simulink library "libreria"  (R2017a)
settings: Solver=VariableStepAuto  StartTime=0.0  StopTime=10.0  RelTol=1e-3
undefined symbols (not defined in the file or in its folder): codertarget, DiscIntNeverNeededParam, gcbh, K, K_PWM, R, Vu, W
libraries: legoev3lib x10, simulink_extras x3, simulink x2
settings Model: Creator=ruben  LastModifiedBy=ruben

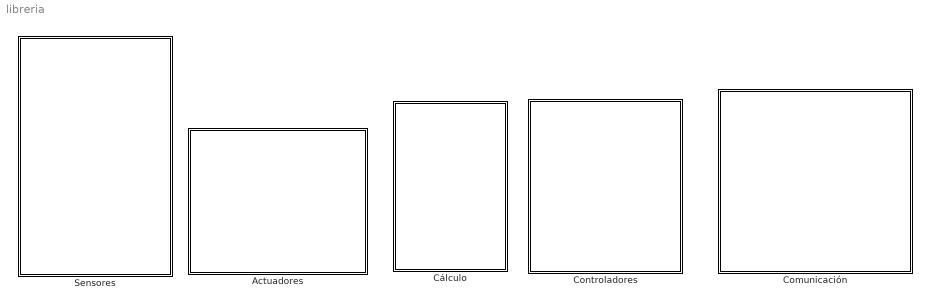
== system libreria ==
  Actuadores : Subsystem
  Comunicación : Subsystem
  Controladores : Subsystem
  Cálculo : Subsystem
  Sensores : Subsystem

== system libreria/Actuadores ==
  Motores : Subsystem  mask(Actuador){}
      mask help:
      | Bloque para la alimentación de los motores en conjunto.
      |
      | Una entrada. Rango de potencia -100/100.
      mask Help:
      | Conexión de entradas:
      | 
      | 	-  Entrada A: Motor izquierdo.
      | 
      | 	- Entrada B: Motor derecho.
      | 
      | Contiene una ganancia para compensar la diferencia existente en la rotación de los motores, explicada en la memoria.
      | 
      | Posibilidad de alimentar cada motor independientemente.
      mask Display: image('D:\RUBEN\Uni\Grado\TFG\Imagenes\Legos\Libreria\motor.png');
  Motores equilibrio : Subsystem  mask(Actuador){}
      mask help:
      | Bloque para la alimentación de los motores en conjunto.
      |
      | Una entrada. Rango de potencia -100/100.
      mask Help:
      | Conexión de entradas:
      | 
      | 	-  Entrada A: Motor izquierdo.
      | 
      | 	- Entrada B: Motor derecho.
      | 
      | Contiene una ganancia para compensar la diferencia existente en la rotación de los motores, explicada en la memoria.
      | 
      | Posibilidad de alimentar cada motor independientemente.
      mask Display: image('D:\RUBEN\Uni\Grado\TFG\Imagenes\Legos\Libreria\motor.png');
  Motores independientes : Subsystem  mask(Actuador){}
      mask help:
      | Bloque para la alimentación de los motores de manera independiente.
      |
      | Dos entradas. Rango de potencia -100/100.
      mask Help:
      | - Puerto A: Motor izquierdo.
      | 
      | - Puerto B: Motor derecho.
      mask Display: image('C:\Users\ruben\Desktop\Eloy\izqu.png');

== system libreria/Comunicación ==
  UDP Envío : S-Function  AncestorBlock=legoev3lib/UDP Send  InitFcn=codertarget.linux.blocks.validateUDPBlock(gcbh);  FunctionName=sdspToNetwork  Parameters=localURL, localPortSource, localPort, remoteURL, remotePort, separateLengthPort, []  SFunctionDeploymentMode=off  EnableBusSupport=off  mask(UDP Envío){remoteURL='127.0.0.1', remotePort=25000, localURL='0.0.0.0', localPortSource=Automatically determine, localPort=2048, sampletime=-1, blockPlatform=LEGO EV3, separateLengthPort=0}
      mask prompts: remoteURL "Dirección IP remota"; remotePort "Puerto IP remoto"; localURL "Dirección IP local"; localPortSource "Fuente Puerto IP local"; localPort "Puerto IP local"; sampletime "Periodo de muestra:"; blockPlatform "Block platform:"; separateLengthPort "Use a separate length port"
      mask help:
      | Envía paquetes UDP a un servidor UDP por medio de una conexión a internet.
      |
      | Establece la dirección IP remota y el puerto IP remoto para realizar la conexión con el servidor.
      mask init:
      | codertarget.linux.blocks.sharedLinuxUDPSendCallback('MaskInitialization');
      mask Help: Para su uso es necesario utilizar el bloque de recepción UDP proporcionado por SIMULINK.
      mask TypeOptions localPortSource: Automatically determine | Specify via dialog
      mask Callback localPortSource:
      | mask_vis = get_param(gcbh, 'MaskVisibilities');
      | if strcmp(get_param(gcbh,'localPortSource'),'Specify via dialog')
      |     mask_vis{5} = 'on';
      | else
      |     mask_vis{5} = 'off';
      | end
      | set_param(gcbh, 'MaskVisibilities', mask_vis);
      | clear('mask_vis');
      mask Display:
      | color('white');
      | plot([100,100,100,100],[100,100,100,100]);
      | plot([0,0,0,0],[0,0,0,0]);
      | color('black');
      | text(0.5, 0.5,'UDP Send\nAddress:127.0.0.1\nPort:25000', 'horizontalAlignment','center','verticalAlignment','middle');
      | color('blue');
      | text(0.90, 0.87, 'LEGO EV3', 'horizontalAlignment', 'right');
  UDP Recepción : S-Function  AncestorBlock=legoev3lib/UDP Receive  InitFcn=codertarget.linux.blocks.validateUDPBlock(gcbh);  FunctionName=sdspFromNetwork  Parameters=localURL, localPort, remoteURL, remotePort, recvBufferSize, signalDatatype, dims, sampletime, isVarSize, blockingTime  SFunctionDeploymentMode=off  EnableBusSupport=off  mask(UDP Receive){localURL='0.0.0.0', localPort=25000, remoteURL='0.0.0.0', remotePort=-1, recvBufferSize=8192, signalDatatype=uint8, dims=255, isVarSize=off, showBlockingTime=off, blockingTime=0, sampletime=0.1, blockPlatform=LEGO EV3}
      mask prompts: localURL "Dirección IP local"; localPort "Puerto IP local"; remoteURL "Dirección IP remota"; remotePort "Puerto IP remoto"; recvBufferSize "Receive buffer size (bytes):"; signalDatatype "Tipo de dato"; dims "Tamaño del dato (N)"; isVarSize "Output variable-size signal"; showBlockingTime "Show blocking time"; blockingTime "Blocking time (seconds):"; sampletime "Periodo de muestreo"; blockPlatform "Block platform:"
      mask help:
      | Recibe paquetes UDP de otro servidor UDP conectado mediante una conexión de internet.
      |
      | La salida del bloque es un array de tamaño [Nx1].
      |
      | Establece el puerto IP local como el número del puerto utilizado en el bloque de envío UDP desde un servidor.
      mask init:
      | codertarget.linux.blocks.sharedLinuxUDPReceiveCallback('MaskInitialization');
      mask Help: Para el uso de este bloque es necesario la utilización del bloque de envío desde un servidor incluido en la librería de Simulink.
      mask TypeOptions signalDatatype: double | single | int8 | uint8 | int16 | uint16 | int32 | uint32 | boolean
      mask Display:
      | color('white');
      | plot([100,100,100,100],[100,100,100,100]);
      | plot([0,0,0,0],[0,0,0,0]);
      | color('black');
      | text(0.5, 0.5,'UDP Send\nPort:25000', 'horizontalAlignment','center','verticalAlignment','middle');
      | color('blue');
      | text(0.90, 0.87, 'LEGO EV3', 'horizontalAlignment', 'right');
      | color('black');
      | port_label('output',1,'Data');
      | port_label('output',2,'Size');

== system libreria/Controladores ==
  Equilibrio : Subsystem  mask(Controlador){}
      mask help: Permite controlar el equilibrio de un robot de morfología inestable.
      mask Display: image('C:\Users\ruben\Desktop\balancingrobots_small1-550x387.jpg');

== system libreria/Cálculo ==
  Odometria : Subsystem  mask(Cálculo){}
      mask help:
      | Permite calcular la posición X Y del robot mediante cálculos de odometría.
      |
      | Una entrada vector de 2 valores. (ENCODER)
      mask Help:
      | Vu=Pi*2*R, definido en el Workspace.
      | 
      | W, definido en el Workspace.
      mask Display: image('D:\RUBEN\Uni\Grado\TFG\Imagenes\Legos\Libreria\odometría.png');
  Theta : Subsystem  mask(Cálculo){}
      mask help:
      | Mediante la información de los encoders, se calcula la posición angular de los motores y su velocidad.
      |
      | Necesaria la ayuda del angulo de inclinación, psi.
      |
      | Dos entradas, psi (valor) y encoders (vector,2).
      mask Help: No es necesaria ninguna variable predefinida.
      mask Display: image('D:\RUBEN\Uni\Grado\TFG\Imagenes\Legos\Libreria\theta.png');
  phi : Subsystem  mask(Cálculo){}
      mask help:
      | Permite calcular, mediante la información de los encoders, tanto la rotación realizada debido al desplazamiento relativo entre las ruedas como la velocidad angular de ese giro.
      |
      | Una entrada de tipo vector de dos valores.
      mask Help:
      | R, radio de la rueda, definido en el Workspace.
      | 
      | W, distancia entre ruedas, definido en el Workspace.
      mask Display: image('D:\RUBEN\Uni\Grado\TFG\Imagenes\Legos\Libreria\phi.png');

== system libreria/Sensores ==
  Color : Subsystem  mask(Sensor){}
      mask help:
      | Diferencia entre 7 colores diferentes y asigna un número a cada uno.
      |
      | Una salida. Tipo Double.
      mask Help:
      | Sensor conectado en el puerto 1.
      | 
      | El periodo de muestreo, Ts, definido en el Workspace.
      | 
      | Asignación de números:
      | 
      | 	-0 No color.
      | 	-1 Negro.
      | 	-2 Azul.
      | 	-3 Verde.
      | 	-4 Amarillo.
      | 	-5 Rojo.
      | 	-6 Blanco.
      | 	-7 Marrón.
      mask Display: image('D:\RUBEN\Uni\Grado\TFG\Imagenes\Legos\color1.png');
  Encoder : Subsystem  mask(Sensor){}
      mask help:
      | Mediante este bloque se conoce la posición angular de los motores.
      |
      | La salida es un vector de 2 valores, una posición para cada encoder. Tipo Double.
      mask Help:
      | La configuración es la siguiente:
      | 
      | 	- Puerto A: Motor izquierdo.
      | 	- Puerto B: Motor derecho.
      | 
      | 	- El medidor no se reinica al alcanzar los 360º.
      | 	- El periodo de muestreo es el utilizado en el resto de prácticas. Ts, definido en el Workspace.
      | 
      | La multiplicación por -1 es utilizada para invertir el sentido de la medida, ya que inicialmente en un avance hacia delante la medida era negativa.
      mask Display: image('D:\RUBEN\Uni\Grado\TFG\Imagenes\Legos\Libreria\partes-encoder.jpg');
  Giroscopo : Subsystem  mask(Sensor){}
      mask help:
      | Mediante este bloque se obtiene la velocidad angular de giro y el angulo girado respecto de un eje.
      |
      | Dos salidas, angulo y velocidad, en radianes. Tipo Double.
      mask Help:
      | El sensor de giro está conectado en el puerto 4.
      | 
      | El periodo de muestreo, Ts, definido en el Workspace.
      mask Display: image('D:\RUBEN\Uni\Grado\TFG\Imagenes\Legos\Libreria\angulo.JPG');
  Ultrasonidos : Subsystem  mask(Sensor){}
      mask help:
      | Determina la distancia entre el robot y elementos del entorno.
      |
      | Una salida en centímetros, rango de medida 0-250cm. Tipo Double.
      mask Help:
      | El sensor está conectado en el puerto 2.
      | 
      | Periodo de muestreo, Ts, definido en el Workspace.
      mask Display: image('D:\RUBEN\Uni\Grado\TFG\Imagenes\Legos\ultra.jpg');

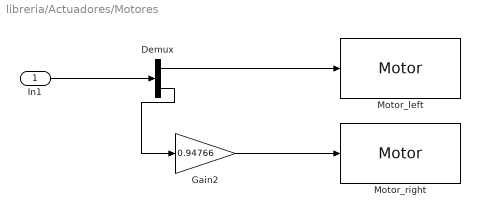
== system libreria/Actuadores/Motores ==
  In1 : Inport
  Demux : Demux  Outputs=2
  Gain2 : Gain  Gain=0.94766
  Motor_left : legoev3lib/Motor  sportNumber=A  sstopAction=Brake
  Motor_right : legoev3lib/Motor  sportNumber=B  sstopAction=Brake
  wires:
  Demux/1 -> Motor_left/1
  Demux/2 -> Gain2/1
  Gain2/1 -> Motor_right/1
  In1/1 -> Demux/1

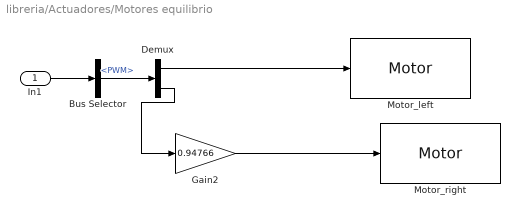
== system libreria/Actuadores/Motores equilibrio ==
  In1 : Inport
  Bus Selector : BusSelector  OutputSignals=PWM
  Demux : Demux  Outputs=2
  Gain2 : Gain  Gain=0.94766
  Motor_left : legoev3lib/Motor  sportNumber=A  sstopAction=Brake
  Motor_right : legoev3lib/Motor  sportNumber=B  sstopAction=Brake
  wires:
  In1/1 -> Bus Selector/1
  Gain2/1 -> Motor_right/1
  Demux/2 -> Gain2/1
  Demux/1 -> Motor_left/1
  Bus Selector/1 -> Demux/1  "<PWM>"

== system libreria/Actuadores/Motores independientes ==
  Mot izq : Inport
  Mot der : Inport  Port=2
  Motor derecho : Subsystem  InitFcn=codertarget.ev3.registry.LEGOvalidateBlock('LEGO MINDSTORMS EV3',gcbh);  mask(LEGO MINDSTORMS EV3 Motor){sportNumber=B, sstopAction=Brake}
      mask prompts: sportNumber "EV3 brick output port:"; sstopAction "Stop action:"
      mask help:
      | Control the power and direction of a motor. The block input accepts integers from 100 to -100:
      | •  100 = Full power forward
      | •    0 = No power
      | • -100 = Full power reverse
      |
      | Select the EV3 brick output port that is connected to this motor.
      mask init:
      | codertarget.ev3.blocks.registerEV3Block(gcbh,'MOTOR');
      | codertarget.ev3.blocks.ev3MotorSysCallback;
      mask Help: eval('codertarget.internal.helpView(''legomindstormsev3'', ''legoev3libev3motor'')')
      mask TypeOptions sportNumber: A | B | C | D
      mask TypeOptions sstopAction: Coast | Brake
      mask Display:
      | iconRoot = codertarget.ev3.blocks.getLEGOEV3BlockIconRoot;
      | iconPath = fullfile(iconRoot, 'motor.gif');
      | [data, map]=imread(iconPath);pic=ind2rgb(data,map);image(pic,[0.32 0.25 0.35 0.55]);
      | switch sportNumber
      |     case 1
      |         text(0.5, 0.15, 'Port A', 'horizontalAlignment', 'center');
      |     case 2
      |         text(0.5, 0.15, 'Port B', 'horizontalAlignment', 'center');
      |     case 3
      |         text(0.5, 0.15, 'Port C', 'horizontalAlignment', 'center');
      |     case 4
      |         text(0.5, 0.15, 'Port D', 'horizontalAlignment', 'center');
      | end
      | port_label('input', 1, '');
      | color('blue');
      | text(0.55, 0.87, 'LEGO EV3', 'horizontalAlignment', 'left');
  Motor izquierdo : legoev3lib/Motor  sportNumber=A  sstopAction=Brake
  wires:
  Mot der/1 -> Motor derecho/1(In1)
  Mot izq/1 -> Motor izquierdo/1

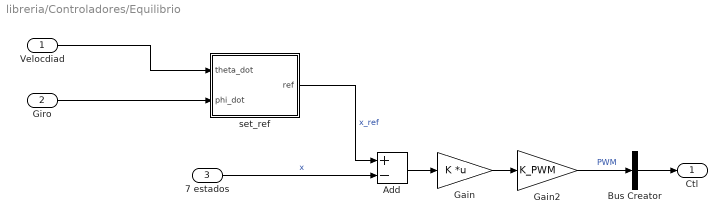
== system libreria/Controladores/Equilibrio ==
  Velocdiad : Inport
  Giro : Inport  Port=2
  7 estados : Inport  Port=3
  Add : Sum  Inputs=+-
  Bus Creator : BusCreator  Inputs=1
  Gain : Gain  Gain=K  Multiplication=Matrix(K*u)
  Gain2 : Gain  Gain=K_PWM
  set_ref : Subsystem
  Ctl : Outport
  wires:
  Gain/1 -> Gain2/1
  Gain2/1 -> Bus Creator/1  "PWM"
  Giro/1 -> set_ref/2(phi_dot)
  Add/1 -> Gain/1
  set_ref/1(ref) -> Add/1  "x_ref"
  7 estados/1 -> Add/2  "x"
  Velocdiad/1 -> set_ref/1(theta_dot)
  Bus Creator/1 -> Ctl/1

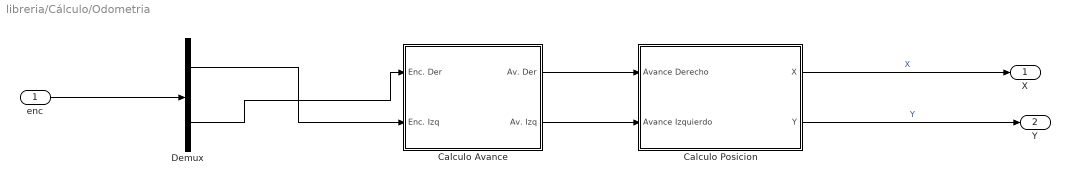
== system libreria/Cálculo/Odometria ==
  enc : Inport
  Calculo Avance : Subsystem
  Calculo Posicion : Subsystem
  Demux : Demux  Outputs=2
  X : Outport
  Y : Outport  Port=2
  wires:
  Calculo Avance/1(Av. Der) -> Calculo Posicion/1("Avance Derecho ")
  Calculo Avance/2(Av. Izq) -> Calculo Posicion/2(Avance Izquierdo)
  Calculo Posicion/2(Y) -> Y/1  "Y"
  Calculo Posicion/1(X) -> X/1  "X"
  enc/1 -> Demux/1
  Demux/1 -> Calculo Avance/2(Enc. Izq)
  Demux/2 -> Calculo Avance/1(Enc. Der)

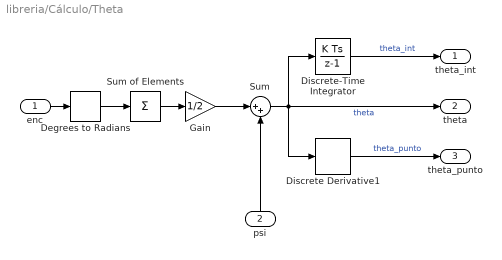
== system libreria/Cálculo/Theta ==
  enc : Inport
  psi : Inport  Port=2
  Degrees to Radians : simulink_extras/Transformations/Degrees to Radians
  Discrete Derivative1 : simulink/Discrete/Discrete Derivative  gainval=1.0  ICPrevScaledInput=0.0  OutMin=[]  OutMax=[]  OutDataType=fixdt(1, 16)  OutScaling=2^-10  DoSatur=off
  Discrete-Time Integrator : DiscreteIntegrator  InitialConditionSetting=State (most efficient)  SampleTime=-1  ICPrevOutput=DiscIntNeverNeededParam  ICPrevScaledInput=DiscIntNeverNeededParam
  Gain : Gain  Gain=1/2
  Sum : Sum  Inputs=|++
  Sum of Elements : Sum  Inputs=+
  theta_int : Outport
  theta : Outport  Port=2
  theta_punto : Outport  Port=3
  wires:
  Degrees to Radians/1 -> Sum of Elements/1
  enc/1 -> Degrees to Radians/1
  Sum of Elements/1 -> Gain/1
  Discrete-Time Integrator/1 -> theta_int/1  "theta_int"
  Gain/1 -> Sum/1
  psi/1 -> Sum/2
  Sum/1 -> theta/1, Discrete-Time Integrator/1, Discrete Derivative1/1  "theta"
  Discrete Derivative1/1 -> theta_punto/1  "theta_punto"

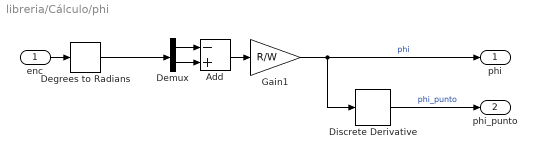
== system libreria/Cálculo/phi ==
  enc : Inport
  Add : Sum  Inputs=-+
  Degrees to Radians : simulink_extras/Transformations/Degrees to Radians
  Demux : Demux  Outputs=2
  Discrete Derivative : simulink/Discrete/Discrete Derivative  gainval=1.0  ICPrevScaledInput=0.0  OutMin=[]  OutMax=[]  OutDataType=fixdt(1, 16)  OutScaling=2^-10  DoSatur=off
  Gain1 : Gain  Gain=R/W
  phi : Outport
  phi_punto : Outport  Port=2
  wires:
  Demux/2 -> Add/2
  Add/1 -> Gain1/1
  Demux/1 -> Add/1
  Gain1/1 -> phi/1, Discrete Derivative/1  "phi"
  Discrete Derivative/1 -> phi_punto/1  "phi_punto"
  Degrees to Radians/1 -> Demux/1
  enc/1 -> Degrees to Radians/1

== system libreria/Sensores/Color ==
  Color Sensor : legoev3lib/Color Sensor  portNumber=1  mode=Color  sampleTime=0.1
      settings: SourceProductName=Simulink Support Package for LEGO MINDSTORMS EV3 Hardware  SourceProductBaseCode=LEGOEV3
  Data Type Conversion1 : DataTypeConversion  OutDataTypeStr=double
  Color : Outport
  wires:
  Color Sensor/1 -> Data Type Conversion1/1
  Data Type Conversion1/1 -> Color/1

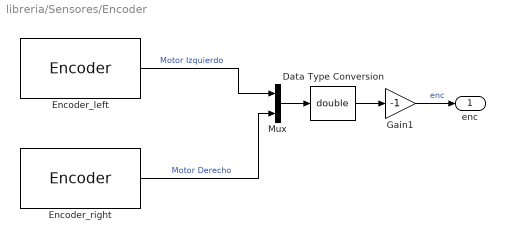
== system libreria/Sensores/Encoder ==
  Data Type Conversion : DataTypeConversion  OutDataTypeStr=double
  Encoder_left : legoev3lib/Encoder  portNumber=A  opMode=No reset  sampleTime=Ts
      settings: SourceProductName=Simulink Support Package for LEGO MINDSTORMS EV3 Hardware  SourceProductBaseCode=LEGOEV3
  Encoder_right : legoev3lib/Encoder  portNumber=B  opMode=No reset  sampleTime=Ts
      settings: SourceProductName=Simulink Support Package for LEGO MINDSTORMS EV3 Hardware  SourceProductBaseCode=LEGOEV3
  Gain1 : Gain  Gain=-1
  Mux : Mux  Inputs=2
  "enc " : Outport
  wires:
  Encoder_left/1 -> Mux/1  "Motor Izquierdo"
  Encoder_right/1 -> Mux/2  "Motor Derecho"
  Data Type Conversion/1 -> Gain1/1
  Mux/1 -> Data Type Conversion/1
  Gain1/1 -> "enc "/1  "enc"

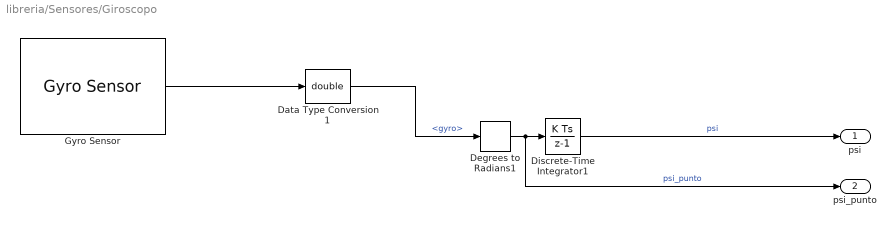
== system libreria/Sensores/Giroscopo ==
  Data Type Conversion1 : DataTypeConversion  OutDataTypeStr=double
  Degrees to Radians1 : simulink_extras/Transformations/Degrees to Radians
  Discrete-Time Integrator1 : DiscreteIntegrator  InitialConditionSetting=State (most efficient)  SampleTime=-1  ICPrevOutput=DiscIntNeverNeededParam  ICPrevScaledInput=DiscIntNeverNeededParam
  Gyro Sensor : legoev3lib/Gyro Sensor  portNumber=4  sampleTime=Ts
      settings: SourceProductName=Simulink Support Package for LEGO MINDSTORMS EV3 Hardware  SourceProductBaseCode=LEGOEV3
  psi : Outport
  psi_punto : Outport  Port=2
  wires:
  Gyro Sensor/1 -> Data Type Conversion1/1
  Discrete-Time Integrator1/1 -> psi/1  "psi"
  Degrees to Radians1/1 -> psi_punto/1, Discrete-Time Integrator1/1  "psi_punto"
  Data Type Conversion1/1 -> Degrees to Radians1/1  "<gyro>"

== system libreria/Sensores/Ultrasonidos ==
  Data Type Conversion1 : DataTypeConversion  OutDataTypeStr=double
  Ultrasonic Sensor : legoev3lib/Ultrasonic Sensor  PortNumber=2  sampleTime=Ts
      settings: SourceProductName=Simulink Support Package for LEGO MINDSTORMS EV3 Hardware  SourceProductBaseCode=LEGOEV3
  Ultrasonidos : Outport
  wires:
  Ultrasonic Sensor/1 -> Data Type Conversion1/1
  Data Type Conversion1/1 -> Ultrasonidos/1

== system libreria/Actuadores/Motores independientes/Motor derecho ==
  In1 : Inport
  Data Type Conversion : DataTypeConversion  OutDataTypeStr=int8  SaturateOnIntegerOverflow=on
  Motor : S-Function  FunctionName=ev3_motor  Parameters=portNumber, stopAction  SFunctionDeploymentMode=off  EnableBusSupport=off  mask(EV3 Motor){portNumber=B, stopAction=Brake}
      mask prompts: portNumber "EV3 Outport Port:"; stopAction "Stop Action:"
      mask help: Sets motor speed and action when stopped.
      mask TypeOptions portNumber: A | B | C | D
      mask TypeOptions stopAction: Coast | Brake
      mask Display:
      | port_label('input', 1, '');
      | color('blue');
      | text(0.45, 0.87, 'LEGO EV3', 'horizontalAlignment', 'left');
  wires:
  In1/1 -> Data Type Conversion/1
  Data Type Conversion/1 -> Motor/1

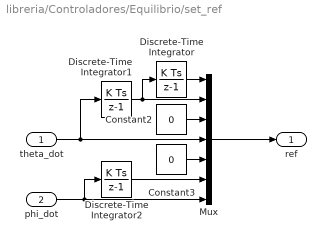
== system libreria/Controladores/Equilibrio/set_ref ==
  theta_dot : Inport
  phi_dot : Inport  Port=2
  Constant2 : Constant  Value=0
  Constant3 : Constant  Value=0
  Discrete-Time Integrator : DiscreteIntegrator  InitialConditionSetting=State (most efficient)  SampleTime=-1  ICPrevOutput=DiscIntNeverNeededParam  ICPrevScaledInput=DiscIntNeverNeededParam
  Discrete-Time Integrator1 : DiscreteIntegrator  InitialConditionSetting=State (most efficient)  SampleTime=-1  ICPrevOutput=DiscIntNeverNeededParam  ICPrevScaledInput=DiscIntNeverNeededParam
  Discrete-Time Integrator2 : DiscreteIntegrator  InitialConditionSetting=State (most efficient)  SampleTime=-1  ICPrevOutput=DiscIntNeverNeededParam  ICPrevScaledInput=DiscIntNeverNeededParam
  Mux : Mux  Inputs=7
  ref : Outport
  wires:
  Constant2/1 -> Mux/3
  Constant3/1 -> Mux/5
  Mux/1 -> ref/1
  Discrete-Time Integrator1/1 -> Discrete-Time Integrator/1, Mux/2
  phi_dot/1 -> Discrete-Time Integrator2/1, Mux/7
  Discrete-Time Integrator2/1 -> Mux/6
  Discrete-Time Integrator/1 -> Mux/1
  theta_dot/1 -> Discrete-Time Integrator1/1, Mux/4

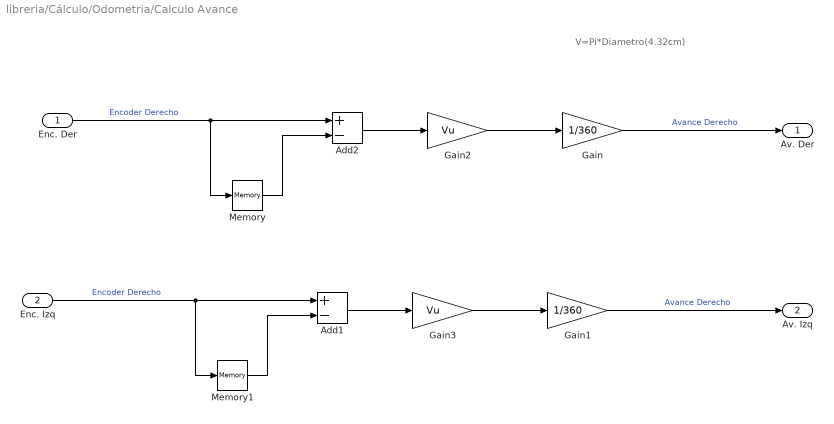
== system libreria/Cálculo/Odometria/Calculo Avance ==
  note: V=Pi*Diametro(4.32cm)
  Enc. Der : Inport
  Enc. Izq : Inport  Port=2
  Add1 : Sum  Inputs=+-
  Add2 : Sum  Inputs=+-
  Gain : Gain  Gain=1/360
  Gain1 : Gain  Gain=1/360
  Gain2 : Gain  Gain=Vu
  Gain3 : Gain  Gain=Vu
  Memory : Memory
  Memory1 : Memory
  Av. Der : Outport
  Av. Izq : Outport  Port=2
  wires:
  Gain/1 -> Av. Der/1  "Avance Derecho"
  Gain2/1 -> Gain/1
  Enc. Der/1 -> Add2/1, Memory/1  "Encoder Derecho"
  Memory/1 -> Add2/2
  Add2/1 -> Gain2/1
  Add1/1 -> Gain3/1
  Memory1/1 -> Add1/2
  Enc. Izq/1 -> Memory1/1, Add1/1  "Encoder Derecho"
  Gain3/1 -> Gain1/1
  Gain1/1 -> Av. Izq/1  "Avance Derecho"

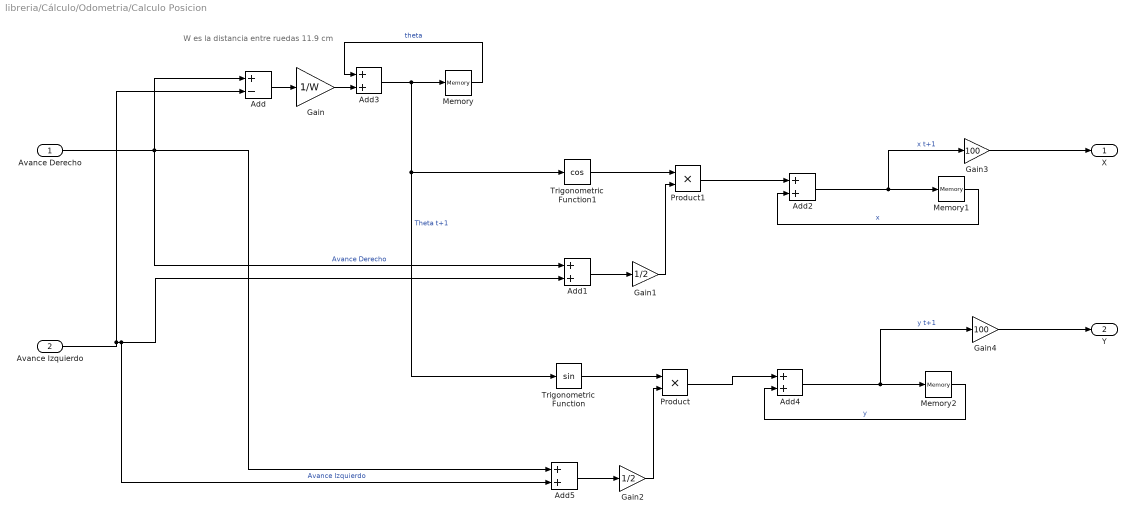
== system libreria/Cálculo/Odometria/Calculo Posicion ==
  note: W es la distancia entre ruedas 11.9 cm
  "Avance Derecho " : Inport
  Avance Izquierdo : Inport  Port=2
  Add : Sum  Inputs=+-
  Add{1..5} (5 alike) : Sum
  Gain : Gain  Gain=1/W
  Gain1 : Gain  Gain=1/2
  Gain2 : Gain  Gain=1/2
  Gain3 : Gain  Gain=100
  Gain4 : Gain  Gain=100
  Memory : Memory
  Memory1 : Memory
  Memory2 : Memory
  Product : Product
  Product1 : Product
  Trigonometric Function : Trigonometry
  Trigonometric Function1 : Trigonometry  Operator=cos
  X : Outport
  Y : Outport  Port=2
  wires:
  Add3/1 -> Trigonometric Function1/1, Trigonometric Function/1, Memory/1  "Theta t+1"
  Add4/1 -> Gain4/1, Memory2/1  "y t+1"
  Memory2/1 -> Add4/2  "y"
  Product/1 -> Add4/1
  Gain/1 -> Add3/2
  Memory/1 -> Add3/1  "theta"
  Trigonometric Function/1 -> Product/1
  Trigonometric Function1/1 -> Product1/1
  Add/1 -> Gain/1
  Add2/1 -> Gain3/1, Memory1/1  "x t+1"
  Product1/1 -> Add2/1
  Gain1/1 -> Product1/2
  Add1/1 -> Gain1/1
  Memory1/1 -> Add2/2  "x"
  "Avance Derecho "/1 -> Add5/1, Add1/1, Add/1  "Avance Derecho"
  Add5/1 -> Gain2/1
  Gain2/1 -> Product/2
  Avance Izquierdo/1 -> Add5/2, Add1/2, Add/2  "Avance Izquierdo"
  Gain3/1 -> X/1
  Gain4/1 -> Y/1
